simulink model "modulador_corriente"  (R2023b)
settings: Solver=VariableStepAuto  StartTime=0.0  StopTime=10.0  RelTol=1e-3
values from neighbouring files (symbols this model uses):
  Ld = 6.6e-3    (= 0.0066)    [constantes.m]
  Lls = 0.8e-3    (= 0.0008)    [constantes.m]
  Lq = 5.8e-3    (= 0.0058)    [constantes.m]
settings Model: Creator=rodri  LastModifiedBy=rodri

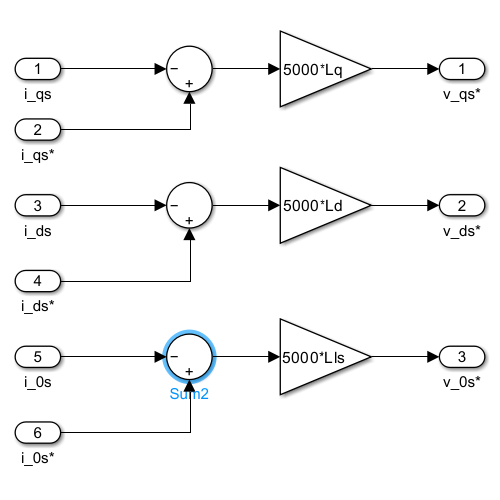
[thumbnail: Simulink's stored preview of the top-level diagram]
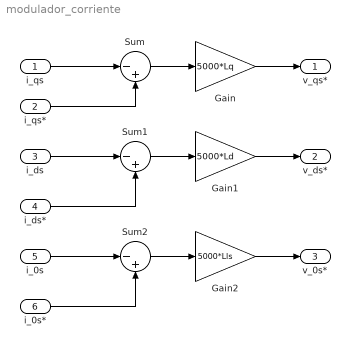
== system modulador_corriente ==
  i_qs : Inport
  i_qs* : Inport  Port=2
  i_ds : Inport  Port=3
  i_ds* : Inport  Port=4
  i_0s : Inport  Port=5
  i_0s* : Inport  Port=6
  Gain : Gain  Gain=5000*Lq
  Gain1 : Gain  Gain=5000*Ld
  Gain2 : Gain  Gain=5000*Lls
  Sum : Sum  Inputs=|-+
  Sum1 : Sum  Inputs=|-+
  Sum2 : Sum  Inputs=|-+
  v_qs* : Outport
  v_ds* : Outport  Port=2
  v_0s* : Outport  Port=3
  wires:
  i_qs/1 -> Sum/1
  i_qs*/1 -> Sum/2
  i_ds/1 -> Sum1/1
  i_ds*/1 -> Sum1/2
  i_0s/1 -> Sum2/1
  i_0s*/1 -> Sum2/2
  Sum/1 -> Gain/1
  Sum1/1 -> Gain1/1
  Sum2/1 -> Gain2/1
  Gain/1 -> v_qs*/1
  Gain1/1 -> v_ds*/1
  Gain2/1 -> v_0s*/1
